simulink model "Tavola3_new"  (R2018b)
settings: Solver=VariableStepAuto  StartTime=0.0  StopTime=10.0  RelTol=1e-3
settings Model: Creator=Utente  LastModifiedBy=Utente

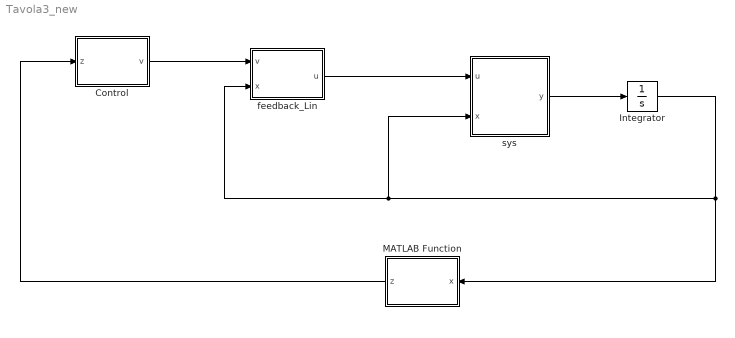
== system Tavola3_new ==
  Control : MATLAB Function  TreatAsAtomicUnit=on
  Integrator : Integrator  InitialCondition=[0;0;0;0;0;5;0]
  MATLAB Function : MATLAB Function  TreatAsAtomicUnit=on
  feedback_Lin : MATLAB Function  TreatAsAtomicUnit=on
  sys : MATLAB Function  TreatAsAtomicUnit=on
  wires:
  sys/1(y) -> Integrator/1
  Integrator/1 -> MATLAB Function/1(x), feedback_Lin/2(x), sys/2(x)
  feedback_Lin/1(u) -> sys/1(u)
  MATLAB Function/1(z) -> Control/1(z)
  Control/1(v) -> feedback_Lin/1(v)

== matlab function Tavola3_new/MATLAB Function ==
  data: x input; z output
function z = coord_trasf(x)         
    
    x1 = x(1);
    x2 = x(2);
    x3 = x(3);
    x4 = x(4);    
    x5 = x(5);
    x6 = x(6);
    x7 = x(7);

    z =  [                                                                                                                                                        x1;
                                                                                                                                                      x6*cos(x3);
             cos(x3)*((1.99*sin(3.0*x4) - 6.77*sin(x4))*x7^2 + (23.5*sin(2.0*x4))/(4.79*cos(x4)^2 - 12.5) - (2.19*x5^2*sin(2.0*x4))/(4.79*cos(x4)^2 - 12.5)) - x6*x7*sin(x3);
                                                                                                                                                              x3;
                                                                                                                                                              x7;
                                                           (0.547*x6*x7*sin(x4))/(0.228*cos(x4)^2 - 0.315) + (0.228*x5*x7*sin(2.0*x4))/(0.228*cos(x4)^2 - 0.315);
                                                                                                                                                             x2];

end

== matlab function Tavola3_new/sys ==
  data: u input; y output; x input
function y = mode_sys(u,x)

    x1 = x(1);
    x2 = x(2);
    x3 = x(3);
    x4 = x(4);    
    x5 = x(5);
    x6 = x(6);
    x7 = x(7);
    
    f = [                                                                                                                         x6*cos(x3);
                                                                                                                                  x6*sin(x3);
                                                                                                                                          x7;
                                                                                                                                          x5;
 (2.39*sin(2.0*x4)*x5^2)/(4.79*cos(x4)^2 - 12.5) - (173.0*sin(x4))/(4.79*cos(x4)^2 - 12.5) - (3.28*x7^2*sin(2.0*x4))/(4.79*cos(x4)^2 - 12.5);
       (1.99*sin(3.0*x4) - 6.77*sin(x4))*x7^2 + (23.5*sin(2.0*x4))/(4.79*cos(x4)^2 - 12.5) - (2.19*x5^2*sin(2.0*x4))/(4.79*cos(x4)^2 - 12.5);
                                       (0.547*x6*x7*sin(x4))/(0.228*cos(x4)^2 - 0.315) + (0.228*x5*x7*sin(2.0*x4))/(0.228*cos(x4)^2 - 0.315)];
                                   
    g1 = [                                                      0;
                                                                0;
                                                                0;
                                                                0;
                    (2.19*cos(x3) + 3.11)/(4.79*cos(x4)^2 - 12.5);
             -(1.0*(0.547*cos(x4) + 1.0))/(4.79*cos(x4)^2 - 12.5);
                                  -0.05/(0.228*cos(x4)^2 - 0.315)];
                  
    g2 = [                                                      0;
                                                                0;
                                                                0;
                                                                0;
                    (2.19*cos(x3) + 3.11)/(4.79*cos(x4)^2 - 12.5);
             -(1.0*(0.547*cos(x4) + 1.0))/(4.79*cos(x4)^2 - 12.5);
                                   0.05/(0.228*cos(x4)^2 - 0.315)];
                   
                   
   y = f+[g1,g2]*u;
   
end

== matlab function Tavola3_new/Control ==
  data: z input; v output
function v = fcn(z)         

    v1 = -k1*(z(1)-setpoint) - k2*(z(2)-d_setpoint);% - k3*(z(3)-d2_setpoint)
    v2 = -k3*(z(3)-setpoint) - k4*(z(4)-d_setpoint);
    
end

== matlab function Tavola3_new/feedback_Lin ==
  data: v input; x input; u output
function u = fcn(v,x)         
    
    x1 = x(1);
    x2 = x(2);
    x3 = x(3);
    x4 = x(4);    
    x5 = x(5);
    x6 = x(6);
    x7 = x(7);

  
    
    
end
